simulink model "Differential_eqn"  (Simulink 9.2)
settings: Solver=ode15s  StartTime=0.0  StopTime=10  RelTol=1e-3  EnableMultiTasking=on
libraries: fl_lib x17, nesl_utility x2
settings Model: Creator=subramanian.krishnan  LastModifiedBy=optiplex3060
settings OptimizationCC: ExpressionDepthLimit=2147483647  InitFltsAndDblsToZero=on
settings SimscapeCC: SimscapeNormalizeSystem=off

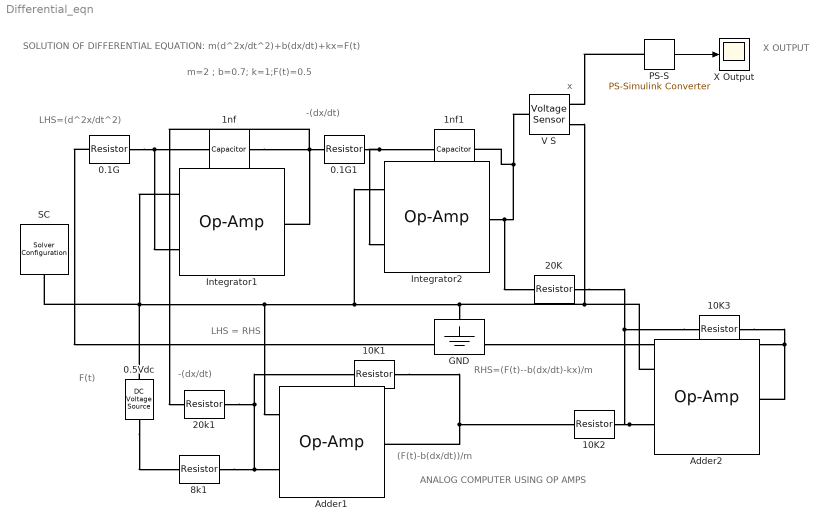
== system Differential_eqn ==
  note: SOLUTION OF DIFFERENTIAL EQUATION: m(d^2x/dt^2)+b(dx/dt)+kx=F(t)
  note: m=2 ; b=0.7; k=1;F(t)=0.5
  note: LHS=(d^2x/dt^2)
  note: -(dx/dt)
  note: x
  note: RHS=(F(t)--b(dx/dt)-kx)/m
  note: LHS = RHS
  note: ANALOG COMPUTER USING OP AMPS
  note: F(t)
  note: -(dx/dt)
  note: (F(t)-b(dx/dt))/m
  note: X OUTPUT
  0.1G : fl_lib/Electrical/Electrical Elements/Resistor  R=0.1 GOhm  i_specify=off  i_priority=None  i=0 A  i_nominal_specify=off  i_nominal_unit=A  i_nominal_value=1  v_specify=off  v_priority=None  v=0 V  v_nominal_specify=off  v_nominal_unit=V  v_nominal_value=1
  0.1G1 : fl_lib/Electrical/Electrical Elements/Resistor  R=0.1 GOhm  i_specify=off  i_priority=None  i=0 A  i_nominal_specify=off  i_nominal_unit=A  i_nominal_value=1  v_specify=off  v_priority=None  v=0 V  v_nominal_specify=off  v_nominal_unit=V  v_nominal_value=1
  0.5Vdc : fl_lib/Electrical/Electrical Sources/DC Voltage Source  v0=0.5 V
  10K1 : fl_lib/Electrical/Electrical Elements/Resistor  R=10 kOhm  i_specify=off  i_priority=None  i=0 A  i_nominal_specify=off  i_nominal_unit=A  i_nominal_value=1  v_specify=off  v_priority=None  v=0 V  v_nominal_specify=off  v_nominal_unit=V  v_nominal_value=1
  10K2 : fl_lib/Electrical/Electrical Elements/Resistor  R=10 kOhm  i_specify=off  i_priority=None  i=0 A  i_nominal_specify=off  i_nominal_unit=A  i_nominal_value=1  v_specify=off  v_priority=None  v=0 V  v_nominal_specify=off  v_nominal_unit=V  v_nominal_value=1
  10K3 : fl_lib/Electrical/Electrical Elements/Resistor  R=10 kOhm  i_specify=off  i_priority=None  i=0 A  i_nominal_specify=off  i_nominal_unit=A  i_nominal_value=1  v_specify=off  v_priority=None  v=0 V  v_nominal_specify=off  v_nominal_unit=V  v_nominal_value=1
  1nf : fl_lib/Electrical/Electrical Elements/Capacitor  c=1e-09 F  r=1e-06 Ohm  g=0 1/Ohm  i_specify=off  i_priority=None  i=0 A  i_nominal_specify=off  i_nominal_unit=A  i_nominal_value=1  v_specify=off  v_priority=None  v=0 V  v_nominal_specify=off  v_nominal_unit=V  v_nominal_value=1  vc_specify=on  vc_priority=High  vc=0 V  vc_nominal_specify=off  vc_nominal_unit=V  vc_nominal_value=1
  1nf1 : fl_lib/Electrical/Electrical Elements/Capacitor  c=1e-09 F  r=1e-06 Ohm  g=0 1/Ohm  i_specify=off  i_priority=None  i=0 A  i_nominal_specify=off  i_nominal_unit=A  i_nominal_value=1  v_specify=off  v_priority=None  v=0 V  v_nominal_specify=off  v_nominal_unit=V  v_nominal_value=1  vc_specify=on  vc_priority=High  vc=0 V  vc_nominal_specify=off  vc_nominal_unit=V  vc_nominal_value=1
  20K : fl_lib/Electrical/Electrical Elements/Resistor  R=20 kOhm  i_specify=off  i_priority=None  i=0 A  i_nominal_specify=off  i_nominal_unit=A  i_nominal_value=1  v_specify=off  v_priority=None  v=0 V  v_nominal_specify=off  v_nominal_unit=V  v_nominal_value=1
  20k1 : fl_lib/Electrical/Electrical Elements/Resistor  R=20 kOhm  i_specify=off  i_priority=None  i=0 A  i_nominal_specify=off  i_nominal_unit=A  i_nominal_value=1  v_specify=off  v_priority=None  v=0 V  v_nominal_specify=off  v_nominal_unit=V  v_nominal_value=1
  8k1 : fl_lib/Electrical/Electrical Elements/Resistor  R=8 kOhm  i_specify=off  i_priority=None  i=0 A  i_nominal_specify=off  i_nominal_unit=A  i_nominal_value=1  v_specify=off  v_priority=None  v=0 V  v_nominal_specify=off  v_nominal_unit=V  v_nominal_value=1
  Adder1 : fl_lib/Electrical/Electrical Elements/Op-Amp  outI_specify=off  outI_priority=None  outI=0 A  outI_nominal_specify=off  outI_nominal_unit=A  outI_nominal_value=1
  Adder2 : fl_lib/Electrical/Electrical Elements/Op-Amp  outI_specify=off  outI_priority=None  outI=0 A  outI_nominal_specify=off  outI_nominal_unit=A  outI_nominal_value=1
  GND : fl_lib/Electrical/Electrical Elements/Electrical Reference
  Integrator1 : fl_lib/Electrical/Electrical Elements/Op-Amp  outI_specify=off  outI_priority=None  outI=0 A  outI_nominal_specify=off  outI_nominal_unit=A  outI_nominal_value=1
  Integrator2 : fl_lib/Electrical/Electrical Elements/Op-Amp  outI_specify=off  outI_priority=None  outI=0 A  outI_nominal_specify=off  outI_nominal_unit=A  outI_nominal_value=1
  PS-S : nesl_utility/PS-Simulink Converter  PhysicalDomain=network_engine_domain  SubClassName=ps_output  LeftPortType=input  RightPortType=output  PseudoPeriodic=off  Frequencies=[]  Unit=1  AffineConversion=off
  SC : nesl_utility/Solver Configuration  PhysicalDomain=network_engine_domain  SubClassName=solver  LeftPortType=input  RightPortType=generic  Tones=[]  Harmonics=[]  SimulateNoise=off  Profile=off  UseLocalSampling=off  EnableSwitchedLinearOptims=on  FrequencyDomain=off  UseCCode=off  RelTol=0.001  AbsTol=1e-06  MinStep=1e-09  ToWorkspace=off  RevertToSquareIcSolve=off  NumHomotopyIterations=100  PhasorMode=off  PhasorModeNumHarmonics=1  DoDC=off  ResidualTolerance=1e-9  UseLocalSolver=off  LocalSolverChoice=NE_BACKWARD_EULER_ADVANCER  LocalSolverSampleTime=.001  DoFixedCost=off  MaxNonlinIter=12  MaxModeIter=2  LinearAlgebra=Sparse  EquationFormulation=NE_TIME_EF  DelaysMemoryBudget=1024  AutomaticFiltering=on  FilteringTimeConstant=0.001  PartitionStorageMethod=AS_NEEDED  PartitionMemoryBudget=1024
  V S : fl_lib/Electrical/Electrical Sensors/Voltage Sensor
  X Output : Scope
  wires:
  PS-S/1 -> X Output/1
  connections:
  Adder2/LConn1 -- V S/RConn2 -- SC/RConn1 -- Integrator1/LConn1 -- 0.5Vdc/RConn1 -- Adder1/LConn1 -- Integrator2/LConn1 -- GND/LConn1
  10K1/RConn1 -- Adder1/RConn1 -- 10K2/LConn1
  PS-S/LConn1 -- V S/RConn1
  0.1G/RConn1 -- Integrator1/LConn2 -- 1nf/LConn1
  Integrator1/RConn1 -- 1nf/RConn1 -- 20k1/LConn1 -- 0.1G1/LConn1
  0.1G1/RConn1 -- 1nf1/LConn1 -- Integrator2/LConn2
  10K3/LConn1 -- 10K2/RConn1 -- Adder2/LConn2 -- 20K/RConn1
  0.1G/LConn1 -- 10K3/RConn1 -- Adder2/RConn1
  8k1/RConn1 -- Adder1/LConn2 -- 10K1/LConn1 -- 20k1/RConn1
  0.5Vdc/LConn1 -- 8k1/LConn1
  Integrator2/RConn1 -- V S/LConn1 -- 1nf1/RConn1 -- 20K/LConn1
